simulink model "traditonal_matlab_zuobiao"  (R2024b)
settings: Solver=FixedStepAuto  StartTime=0.0  StopTime=1  FixedStep=1e-5  RelTol=1e-3
settings Model: Creator=罗芳成  LastModifiedBy=罗芳成

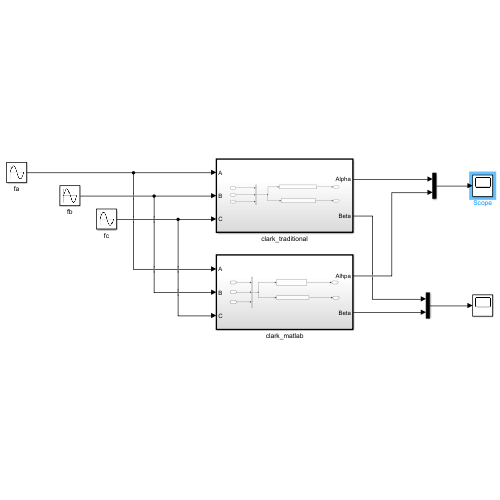
[thumbnail: Simulink's stored preview of the top-level diagram]
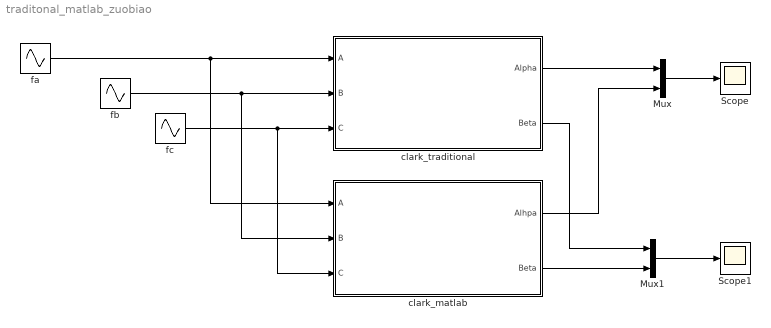
== system traditonal_matlab_zuobiao ==
  Mux : Mux  Inputs=2
  Mux1 : Mux  Inputs=2
  Scope : Scope
  Scope1 : Scope
  clark_matlab : Subsystem  TreatAsAtomicUnit=on
  clark_traditional : Subsystem  TreatAsAtomicUnit=on
  fa : Sin  Amplitude=100  Frequency=100*pi  SampleTime=0
  fb : Sin  Amplitude=100  Frequency=100*pi  Phase=-2*pi/3  SampleTime=0
  fc : Sin  Amplitude=100  Frequency=100*pi  Phase=2*pi/3  SampleTime=0
  wires:
  fa/1 -> clark_traditional/1(A), clark_matlab/1(A)
  fb/1 -> clark_matlab/2(B), clark_traditional/2(B)
  fc/1 -> clark_matlab/3(C), clark_traditional/3(C)
  clark_matlab/1(Alhpa) -> Mux/2
  clark_traditional/1(Alpha) -> Mux/1
  clark_traditional/2(Beta) -> Mux1/1
  clark_matlab/2(Beta) -> Mux1/2
  Mux/1 -> Scope/1
  Mux1/1 -> Scope1/1

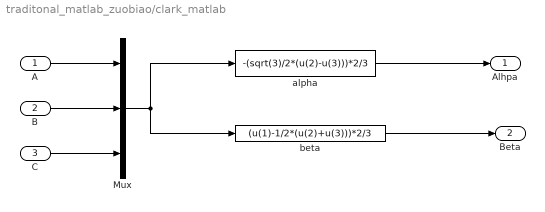
== system traditonal_matlab_zuobiao/clark_matlab ==
  A : Inport
  B : Inport  Port=2
  C : Inport  Port=3
  Mux : Mux  Inputs=3
  alpha : Fcn  Expr=-(sqrt(3)/2*(u(2)-u(3)))*2/3
  beta : Fcn  Expr=(u(1)-1/2*(u(2)+u(3)))*2/3
  Alhpa : Outport
  Beta : Outport  Port=2
  wires:
  A/1 -> Mux/1
  B/1 -> Mux/2
  C/1 -> Mux/3
  Mux/1 -> beta/1, alpha/1
  beta/1 -> Beta/1
  alpha/1 -> Alhpa/1

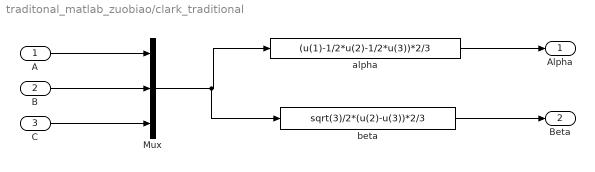
== system traditonal_matlab_zuobiao/clark_traditional ==
  A : Inport
  B : Inport  Port=2
  C : Inport  Port=3
  Mux : Mux  Inputs=3
  alpha : Fcn  Expr=(u(1)-1/2*u(2)-1/2*u(3))*2/3
  beta : Fcn  Expr=sqrt(3)/2*(u(2)-u(3))*2/3
  Alpha : Outport
  Beta : Outport  Port=2
  wires:
  A/1 -> Mux/1
  B/1 -> Mux/2
  C/1 -> Mux/3
  Mux/1 -> beta/1, alpha/1
  beta/1 -> Beta/1
  alpha/1 -> Alpha/1
